simulink model "Spindle_Speed_Control_Loop_simulink"  (R2024b)
settings: Solver=ode4  StartTime=0.0  StopTime=0.3  FixedStep=0.0001  RelTol=1e-3
libraries: slpidlib x1
settings Model: Creator=zahir  LastModifiedBy=zahir
settings DataIOCC: SaveOutput=off  SaveTime=off

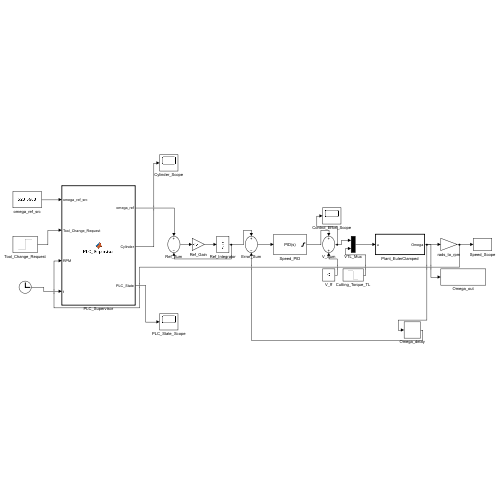
[thumbnail: Simulink's stored preview of the top-level diagram]
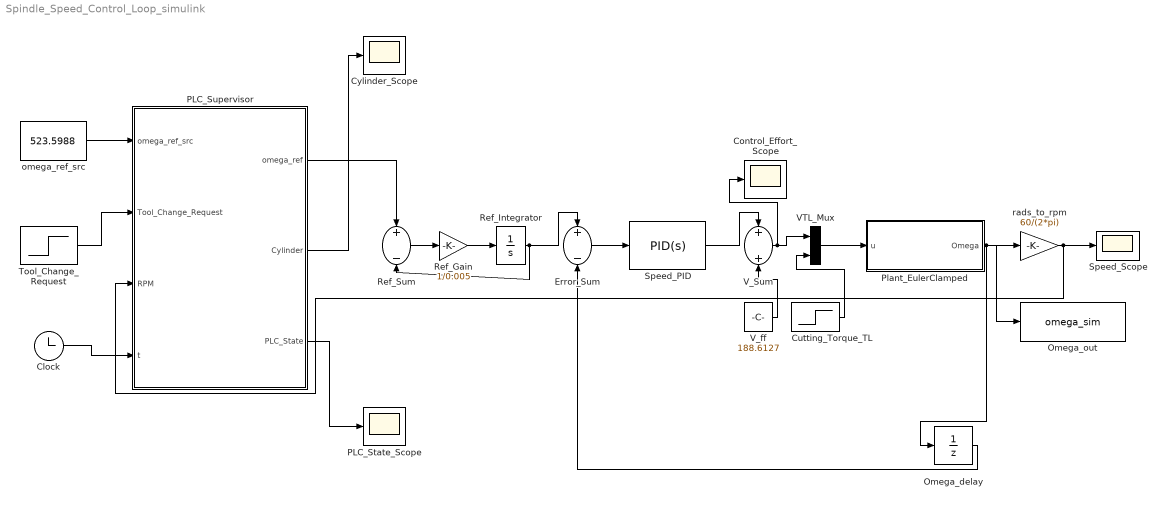
== system Spindle_Speed_Control_Loop_simulink ==
  Clock : Clock
  Control_Effort_Scope : Scope
  Cutting_Torque_TL : Step  Time=0.1  Before=0.675  After=0  SampleTime=0
  Cylinder_Scope : Scope
  Error_Sum : Sum  Inputs=+-
  Omega_delay : UnitDelay  InitialCondition=523.5988  SampleTime=0.0001  HasFrameUpgradeWarning=on
  Omega_out : ToWorkspace  VariableName=omega_sim  SaveFormat=Structure With Time  SampleTime=-1
  PLC_State_Scope : Scope
  PLC_Supervisor : MATLAB Function  TreatAsAtomicUnit=on
  Plant_EulerClamped : MATLAB Function  TreatAsAtomicUnit=on
  Ref_Gain : Gain  Gain=1/0.005
  Ref_Integrator : Integrator  InitialCondition=523.5988
  Ref_Sum : Sum  Inputs=+-
  Speed_PID : slpidlib/PID Controller  Controller=PID  Form=Parallel  TimeDomain=Continuous-time  UseExternalTs=off  SampleTime=-1  IntegratorMethod=Forward Euler  FilterMethod=Forward Euler  ControllerParametersSource=internal  P=0.6118  I=66.96  UseKiTs=off  D=0.00385  UseExternalDerivativeSource=off  N=1000  UseFilter=on  TunerSelectOption=Transfer Function Based (PID Tuner App)  InitialConditionSource=internal  InitialConditionForIntegrator=0  InitialConditionForFilter=0  DifferentiatorICPrevScaledInput=0  ExternalReset=none  TrackingMode=off  Kt=1  LimitOutput=on  SatLimitsSource=internal  UpperSaturationLimit=325  LowerSaturationLimit=-325  LinearizeAsGain=on  AntiWindupMode=clamping  Kb=1  LimitIntegrator=off  UpperIntegratorSaturationLimit=inf  LowerIntegratorSaturationLimit=-inf  POutMin=[]  POutMax=[]  IOutMin=[]  IOutMax=[]  DOutMin=[]  DOutMax=[]  NOutMin=[]  NOutMax=[]  SumOutMin=[]  SumOutMax=[]  SaturationOutMin=[]  SaturationOutMax=[]  PParamMin=[]  PParamMax=[]  IParamMin=[]  IParamMax=[]  DParamMin=[]  DParamMax=[]  NParamMin=[]  NParamMax=[]  KbParamMin=[]  KbParamMax=[]  KtParamMin=[]  KtParamMax=[]  KbOutMin=[]  KbOutMax=[]  KtOutMin=[]  KtOutMax=[]  IntegratorOutMin=[]  IntegratorOutMax=[]  FilterOutMin=[]  FilterOutMax=[]  SumI1OutMin=[]  SumI1OutMax=[]  SumI2OutMin=[]  SumI2OutMax=[]  SumI3OutMin=[]  SumI3OutMax=[]  SumI4OutMin=[]  SumI4OutMax=[]  SumDOutMin=[]  SumDOutMax=[]  DifferentiatorOutMin=[]  DifferentiatorOutMax=[]  FilterDiffOutCoefMin=[]  FilterDiffOutCoefMax=[]  ReciprocalOutMin=[]  ReciprocalOutMax=[]  SumDenOutMin=[]  SumDenOutMax=[]  SumNumOutMin=[]  SumNumOutMax=[]  DivideOutMin=[]  DivideOutMax=[]  UdiffTsProdOutMin=[]  UdiffTsProdOutMax=[]  NTsProdOutMin=[]  NTsProdOutMax=[]  UintegralTsProdOutMin=[]  UintegralTsProdOutMax=[]  UngainTsProdOutMin=[]  UngainTsProdOutMax=[]  ClampingZeroOutDataTypeStr=Inherit: Inherit via back propagation  ClampingZeroOutMin=[]  ClampingZeroOutMax=[]  FilterDenConstantOutDataTypeStr=Inherit: Inherit via back propagation  FilterDenConstantOutMin=[]  FilterDenConstantOutMax=[]  PCopyOutDataTypeStr=Inherit: Inherit via back propagation  PCopyOutMin=[]  PCopyOutMax=[]  NCopyOutDataTypeStr=Inherit: Inherit via back propagation  NCopyOutMin=[]  NCopyOutMax=[]  IntegratorContinuousStateAttributes=''  IntegratorStateMustResolveToSignalObject=off  IntegratorRTWStateStorageClass=Auto  FilterContinuousStateAttributes=''  FilterStateMustResolveToSignalObject=off  FilterRTWStateStorageClass=Auto  ParallelPVariant=InternalParameters  IdealPVariant=Disabled  IVariant=InternalParameters  DVariant=InternalParameters  IntegratorVariant=Continuous  SatVariant=Enabled  AWVariant=ContClampingParallel  PCopyVariant=Disabled  TRVariant=Disabled  FdbkBlocksVariant=Forward  IdealPFdbkVariant=Disabled  SatFdbkVariant=Disabled  DerivativeFilterVariant=ContFilter  NVariant=InternalParameters  NCopyVariant=Disabled  FilterICVariant=InternalICsFilter  IntegratorICVariant=InternalICs  ExternalResetVariant=Disabled  TRSumVariant=Passthrough  SumFdbkVariant=Disabled  SumVariant=Sum_PID  TsampFilterVariant=InternalTs  TsampNgainVariant=Passthrough  TsampIntegralVariant=Disabled_SignalSpec  ExternalSaturationOutDataTypeStr=Inherit: Same as second input  DerivativeSourceVariant=ErrorSignal  PreIntVariant=InternalPreInt
  Speed_Scope : Scope
  Tool_Change_Request : Step  Time=0.1  SampleTime=0
  VTL_Mux : Mux  Inputs=2
  V_Sum : Sum
  V_ff : Constant  Value=188.6127
  omega_ref_src : Constant  Value=523.5988
  rads_to_rpm : Gain  Gain=60/(2*pi)
  wires:
  omega_ref_src/1 -> PLC_Supervisor/1(omega_ref_src)
  Tool_Change_Request/1 -> PLC_Supervisor/2(Tool_Change_Request)
  Clock/1 -> PLC_Supervisor/4(t)
  PLC_Supervisor/1(omega_ref) -> Ref_Sum/1
  Ref_Sum/1 -> Ref_Gain/1
  Ref_Gain/1 -> Ref_Integrator/1
  Ref_Integrator/1 -> Ref_Sum/2, Error_Sum/1
  Error_Sum/1 -> Speed_PID/1
  Speed_PID/1 -> V_Sum/1
  V_ff/1 -> V_Sum/2
  V_Sum/1 -> Control_Effort_Scope/1, VTL_Mux/1
  Cutting_Torque_TL/1 -> VTL_Mux/2
  VTL_Mux/1 -> Plant_EulerClamped/1(u)
  Plant_EulerClamped/1(Omega) -> rads_to_rpm/1, Omega_out/1, Omega_delay/1
  rads_to_rpm/1 -> Speed_Scope/1, PLC_Supervisor/3(RPM)
  PLC_Supervisor/2(Cylinder) -> Cylinder_Scope/1
  PLC_Supervisor/3(PLC_State) -> PLC_State_Scope/1
  Omega_delay/1 -> Error_Sum/2

== matlab function Spindle_Speed_Control_Loop_simulink/Plant_EulerClamped ==
  settings: updateMethod=DISCRETE  sampleTime=0.0001
  data: u input; Omega output
function Omega = Plant_EulerClamped(u)
%#codegen
% u = [V; TL]  from the Mux.
% Output is computed FIRST from the old persistent state, then the
% state is advanced -- this keeps the algebraic character of the
% block as clean as possible.  The real loop-breaker in this model
% is the Unit Delay block on the feedback path.

Omega = 0;                    % explicit scalar output size
persistent x
if isempty(x)
    Jp = 5.45e-4;  Bp = 5.00e-4;
    Rp = 2.0;      Lp = 0.008;
    Ktp = 0.35;    Kep = 0.35;
    omega_nom_p  = 5000 * 2*pi/60;
    TL_nominal_p = 0.675;
    I_ss_p       = (Bp*omega_nom_p + TL_nominal_p)/Ktp;
    x = [I_ss_p; omega_nom_p];
end

% ---- output from previous state ---------------------------------
Omega = x(2);

% ---- Euler update using current input ---------------------------
dt = 1e-4;
Jp = 5.45e-4;  Bp = 5.00e-4;
Rp = 2.0;      Lp = 0.008;
Ktp = 0.35;    Kep = 0.35;
Ap  = [-Rp/Lp, -Kep/Lp; Ktp/Jp, -Bp/Jp];
Bp2 = [1/Lp, 0; 0, -1/Jp];
dx = Ap*x + Bp2*u;
x  = x + dx*dt;
if x(2) < 0
    x(2) = 0;
end
end

== matlab function Spindle_Speed_Control_Loop_simulink/PLC_Supervisor ==
  settings: updateMethod=DISCRETE  sampleTime=0.0001
  data: omega_ref_src input; omega_ref output; Tool_Change_Request input; RPM input; t input; Cylinder output; PLC_State output
function [omega_ref, Cylinder, PLC_State] = PLC_Supervisor(omega_ref_src, Tool_Change_Request, RPM, t)
%#codegen
persistent state release_timer
if isempty(state), state = 0; release_timer = 0; end
RPM_stop_threshold = 5;
release_delay      = 0.020;
omega_ref = 0;  Cylinder = 0;
if Tool_Change_Request == 0
    state = 0;
else
    switch state
        case 0, state = 1;
        case 1
            if abs(RPM) <= RPM_stop_threshold
                state = 2; release_timer = t;
            end
        case 2
            if abs(RPM) > RPM_stop_threshold
                state = 1; release_timer = 0;
            elseif (t - release_timer) >= release_delay
                Cylinder = 1; state = 3;
            end
        case 3, Cylinder = 1;
    end
end
if state == 0
    omega_ref = omega_ref_src;
else
    omega_ref = 0;
end
PLC_State = state;
end
